simulink model "panelMotor_data_control_2018"  (R2018a)
settings: Solver=VariableStepAuto  StartTime=0.0  StopTime=15*3600  RelTol=1e-3
values from neighbouring files (symbols this model uses):
  J = m/12*(l^2*cos(beta)^2+d^2*sin(beta)^2+w^2)    [panelMotorParams.m]
  Jp = m/12*(w^2*cos(beta)^2+d^2*sin(beta)^2+l^2)    [panelMotorParams.m]
  Kd = 5    [panelMotorParams.m]
  Kf = 0.07    [panelMotorParams.m]
  Kg = 2000    [panelMotorParams.m]
  Kt = 0.07    [panelMotorParams.m]
  L = 1e-5    (= 1e-05)    [panelMotorParams.m]
  R = 10    [panelMotorParams.m]
libraries: simulink x3
settings Model: Creator=goku-ubuntu  LastModifiedBy=goku-ubuntu
settings DataIOCC: ExternalInput=[sunTime, sunPosition, sunElevation]  LoadExternalInput=on

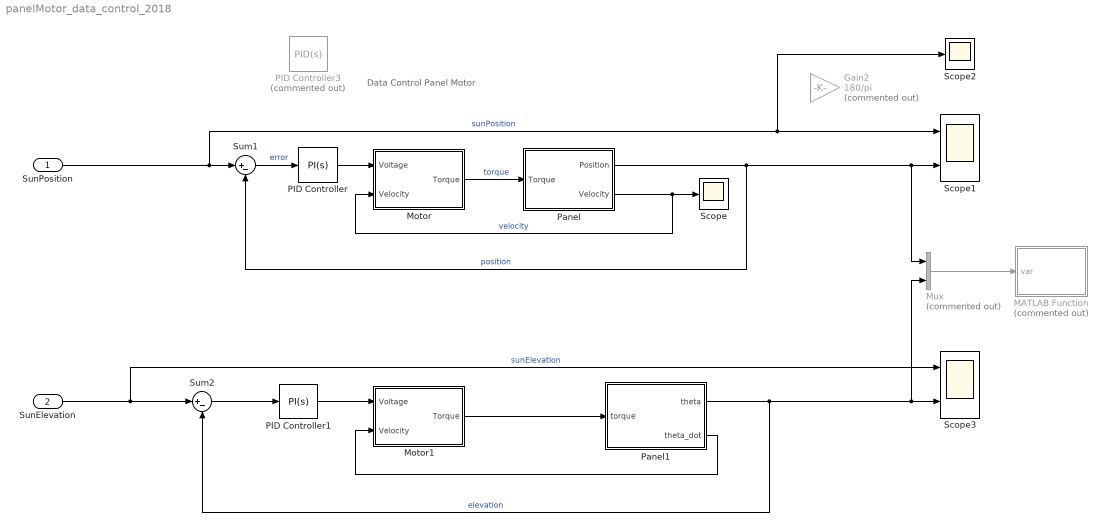
== system panelMotor_data_control_2018 ==
  note: Data Control Panel Motor
  SunPosition : Inport
  SunElevation : Inport  Port=2
  Gain2 : Gain  Commented=on  Gain=180/pi
  MATLAB Function : MATLAB Function  Commented=on  TreatAsAtomicUnit=on
  Motor : Subsystem
  Motor1 : Subsystem
  Mux : Mux  Commented=on  Inputs=2
  PID Controller : simulink/Continuous/PID Controller  Controller=PI  TimeDomain=Continuous-time  SampleTime=-1  IntegratorMethod=Forward Euler  FilterMethod=Forward Euler  Form=Parallel  UseFilter=on  ControllerParametersSource=internal  P=240  I=180  D=0  N=100  InitialConditionSource=internal  InitialConditionForIntegrator=0  InitialConditionForFilter=0  ExternalReset=none  LimitOutput=off  UpperSaturationLimit=inf  LowerSaturationLimit=-inf  LinearizeAsGain=on  AntiWindupMode=none  Kb=1  TrackingMode=off  Kt=1  PParamMin=[]  PParamMax=[]  IParamMin=[]  IParamMax=[]  DParamMin=[]  DParamMax=[]  NParamMin=[]  NParamMax=[]  KbParamMin=[]  KbParamMax=[]  KtParamMin=[]  KtParamMax=[]  POutMin=[]  POutMax=[]  IOutMin=[]  IOutMax=[]  DOutMin=[]  DOutMax=[]  NOutMin=[]  NOutMax=[]  KbOutMin=[]  KbOutMax=[]  KtOutMin=[]  KtOutMax=[]  IntegratorOutMin=[]  IntegratorOutMax=[]  FilterOutMin=[]  FilterOutMax=[]  SumOutMin=[]  SumOutMax=[]  SumI1OutMin=[]  SumI1OutMax=[]  SumI2OutMin=[]  SumI2OutMax=[]  SumI3OutMin=[]  SumI3OutMax=[]  SumDOutMin=[]  SumDOutMax=[]  SaturationOutMin=[]  SaturationOutMax=[]  IntegratorContinuousStateAttributes=''  IntegratorStateMustResolveToSignalObject=off  IntegratorRTWStateStorageClass=Auto  FilterContinuousStateAttributes=''  FilterStateMustResolveToSignalObject=off  FilterRTWStateStorageClass=Auto  DifferentiatorICPrevScaledInput=0  DifferentiatorOutMin=[]  DifferentiatorOutMax=[]  FilterDiffOutCoefMin=[]  FilterDiffOutCoefMax=[]  SumDenOutMin=[]  SumDenOutMax=[]  SumNumOutMin=[]  SumNumOutMax=[]  ReciprocalOutMin=[]  ReciprocalOutMax=[]  DivideOutMin=[]  DivideOutMax=[]  TunerSelectOption=Transfer Function Based (PID Tuner App)
  PID Controller1 : simulink/Continuous/PID Controller  Controller=PI  TimeDomain=Continuous-time  SampleTime=-1  IntegratorMethod=Forward Euler  FilterMethod=Forward Euler  Form=Parallel  UseFilter=on  ControllerParametersSource=internal  P=8839.69591986541  I=114833.219838399  D=0  N=100  InitialConditionSource=internal  InitialConditionForIntegrator=0  InitialConditionForFilter=0  ExternalReset=none  LimitOutput=off  UpperSaturationLimit=inf  LowerSaturationLimit=-inf  LinearizeAsGain=on  AntiWindupMode=none  Kb=1  TrackingMode=off  Kt=1  PParamMin=[]  PParamMax=[]  IParamMin=[]  IParamMax=[]  DParamMin=[]  DParamMax=[]  NParamMin=[]  NParamMax=[]  KbParamMin=[]  KbParamMax=[]  KtParamMin=[]  KtParamMax=[]  POutMin=[]  POutMax=[]  IOutMin=[]  IOutMax=[]  DOutMin=[]  DOutMax=[]  NOutMin=[]  NOutMax=[]  KbOutMin=[]  KbOutMax=[]  KtOutMin=[]  KtOutMax=[]  IntegratorOutMin=[]  IntegratorOutMax=[]  FilterOutMin=[]  FilterOutMax=[]  SumOutMin=[]  SumOutMax=[]  SumI1OutMin=[]  SumI1OutMax=[]  SumI2OutMin=[]  SumI2OutMax=[]  SumI3OutMin=[]  SumI3OutMax=[]  SumDOutMin=[]  SumDOutMax=[]  SaturationOutMin=[]  SaturationOutMax=[]  IntegratorContinuousStateAttributes=''  IntegratorStateMustResolveToSignalObject=off  IntegratorRTWStateStorageClass=Auto  FilterContinuousStateAttributes=''  FilterStateMustResolveToSignalObject=off  FilterRTWStateStorageClass=Auto  DifferentiatorICPrevScaledInput=0  DifferentiatorOutMin=[]  DifferentiatorOutMax=[]  FilterDiffOutCoefMin=[]  FilterDiffOutCoefMax=[]  SumDenOutMin=[]  SumDenOutMax=[]  SumNumOutMin=[]  SumNumOutMax=[]  ReciprocalOutMin=[]  ReciprocalOutMax=[]  DivideOutMin=[]  DivideOutMax=[]  TunerSelectOption=Transfer Function Based (PID Tuner App)
  PID Controller3 : simulink/Continuous/PID Controller  Commented=on  Controller=PID  TimeDomain=Continuous-time  SampleTime=-1  IntegratorMethod=Forward Euler  FilterMethod=Forward Euler  Form=Parallel  UseFilter=on  ControllerParametersSource=internal  P=65852.2280611086  I=3527604.18786694  D=217.337883352011  N=1464.14190878137  InitialConditionSource=internal  InitialConditionForIntegrator=0  InitialConditionForFilter=0  ExternalReset=none  LimitOutput=off  UpperSaturationLimit=inf  LowerSaturationLimit=-inf  LinearizeAsGain=on  AntiWindupMode=none  Kb=1  TrackingMode=off  Kt=1  PParamMin=[]  PParamMax=[]  IParamMin=[]  IParamMax=[]  DParamMin=[]  DParamMax=[]  NParamMin=[]  NParamMax=[]  KbParamMin=[]  KbParamMax=[]  KtParamMin=[]  KtParamMax=[]  POutMin=[]  POutMax=[]  IOutMin=[]  IOutMax=[]  DOutMin=[]  DOutMax=[]  NOutMin=[]  NOutMax=[]  KbOutMin=[]  KbOutMax=[]  KtOutMin=[]  KtOutMax=[]  IntegratorOutMin=[]  IntegratorOutMax=[]  FilterOutMin=[]  FilterOutMax=[]  SumOutMin=[]  SumOutMax=[]  SumI1OutMin=[]  SumI1OutMax=[]  SumI2OutMin=[]  SumI2OutMax=[]  SumI3OutMin=[]  SumI3OutMax=[]  SumDOutMin=[]  SumDOutMax=[]  SaturationOutMin=[]  SaturationOutMax=[]  IntegratorContinuousStateAttributes=''  IntegratorStateMustResolveToSignalObject=off  IntegratorRTWStateStorageClass=Auto  FilterContinuousStateAttributes=''  FilterStateMustResolveToSignalObject=off  FilterRTWStateStorageClass=Auto  DifferentiatorICPrevScaledInput=0  DifferentiatorOutMin=[]  DifferentiatorOutMax=[]  FilterDiffOutCoefMin=[]  FilterDiffOutCoefMax=[]  SumDenOutMin=[]  SumDenOutMax=[]  SumNumOutMin=[]  SumNumOutMax=[]  ReciprocalOutMin=[]  ReciprocalOutMax=[]  DivideOutMin=[]  DivideOutMax=[]  TunerSelectOption=Transfer Function Based (PID Tuner App)
  Panel : Subsystem
  Panel1 : Subsystem
  Scope : Scope
  Scope1 : Scope  NumInputPorts=2
  Scope2 : Scope
  Scope3 : Scope  NumInputPorts=2
  Sum1 : Sum  Inputs=|+-
  Sum2 : Sum  Inputs=|+-
  wires:
  Panel/2(Velocity) -> Motor/2(Velocity), Scope/1  "velocity"
  Panel/1(Position) -> Sum1/2, Mux/1, Scope1/2  "position"
  Motor/1(Torque) -> Panel/1(Torque)  "torque"
  Sum1/1 -> PID Controller/1  "error"
  PID Controller/1 -> Motor/1(Voltage)
  SunPosition/1 -> Sum1/1, Scope1/1, Scope2/1  "sunPosition"
  Motor1/1(Torque) -> Panel1/1(torque)
  Panel1/2(theta_dot) -> Motor1/2(Velocity)
  Panel1/1(theta) -> Sum2/2, Mux/2, Scope3/2  "elevation"
  PID Controller1/1 -> Motor1/1(Voltage)
  Sum2/1 -> PID Controller1/1
  SunElevation/1 -> Sum2/1, Scope3/1  "sunElevation"
  Mux/1 -> MATLAB Function/1(var)

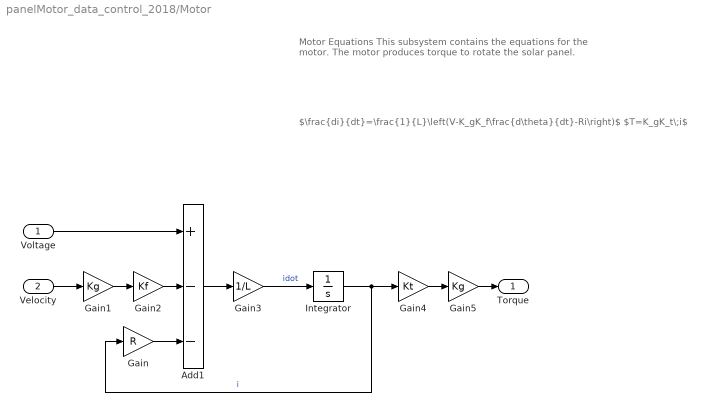
== system panelMotor_data_control_2018/Motor ==
  note: $\frac{di}{dt}=\frac{1}{L}\left(V-K_gK_f\frac{d\theta}{dt}-Ri\right)$
      | $T=K_gK_t\;i$
  note: Motor Equations
      |
      | This subsystem contains the equations for the motor. The motor produces torque to rotate the solar panel.
  Voltage : Inport
  Velocity : Inport  Port=2
  Add1 : Sum  Inputs=+--
  Gain : Gain  Gain=R
  Gain1 : Gain  Gain=Kg
  Gain2 : Gain  Gain=Kf
  Gain3 : Gain  Gain=1/L
  Gain4 : Gain  Gain=Kt
  Gain5 : Gain  Gain=Kg
  Integrator : Integrator
  Torque : Outport  VectorParamsAs1DForOutWhenUnconnected=on
  wires:
  Voltage/1 -> Add1/1
  Gain2/1 -> Add1/2
  Gain3/1 -> Integrator/1  "idot"
  Gain/1 -> Add1/3
  Integrator/1 -> Gain4/1, Gain/1  "i"
  Add1/1 -> Gain3/1
  Velocity/1 -> Gain1/1
  Gain4/1 -> Gain5/1
  Gain1/1 -> Gain2/1
  Gain5/1 -> Torque/1

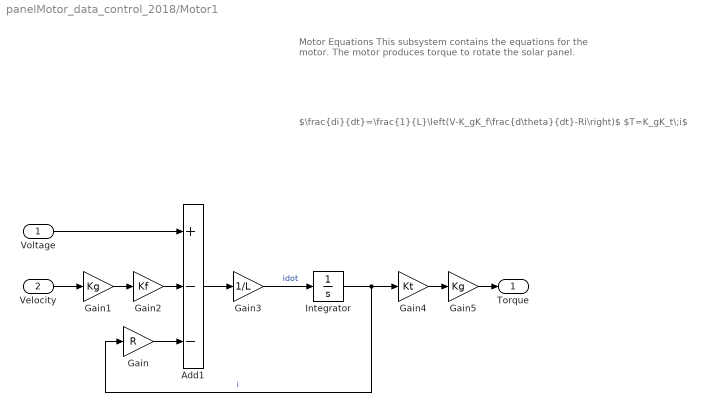
== system panelMotor_data_control_2018/Motor1 ==
  note: Motor Equations
      |
      | This subsystem contains the equations for the motor. The motor produces torque to rotate the solar panel.
  note: $\frac{di}{dt}=\frac{1}{L}\left(V-K_gK_f\frac{d\theta}{dt}-Ri\right)$
      | $T=K_gK_t\;i$
  Voltage : Inport
  Velocity : Inport  Port=2
  Add1 : Sum  Inputs=+--
  Gain : Gain  Gain=R
  Gain1 : Gain  Gain=Kg
  Gain2 : Gain  Gain=Kf
  Gain3 : Gain  Gain=1/L
  Gain4 : Gain  Gain=Kt
  Gain5 : Gain  Gain=Kg
  Integrator : Integrator
  Torque : Outport  VectorParamsAs1DForOutWhenUnconnected=on
  wires:
  Gain5/1 -> Torque/1
  Gain1/1 -> Gain2/1
  Gain4/1 -> Gain5/1
  Velocity/1 -> Gain1/1
  Add1/1 -> Gain3/1
  Integrator/1 -> Gain/1, Gain4/1  "i"
  Gain/1 -> Add1/3
  Gain3/1 -> Integrator/1  "idot"
  Gain2/1 -> Add1/2
  Voltage/1 -> Add1/1

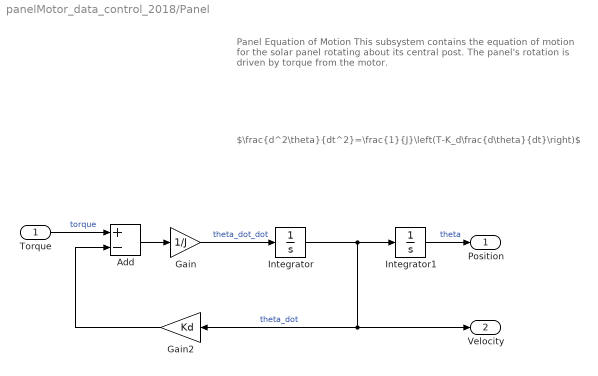
== system panelMotor_data_control_2018/Panel ==
  note: $\frac{d^2\theta}{dt^2}=\frac{1}{J}\left(T-K_d\frac{d\theta}{dt}\right)$
  note: Panel Equation of Motion
      |
      | This subsystem contains the equation of motion for the solar panel rotating about its central post. The panel's rotation is driven by torque from the motor.
  Torque : Inport
  Add : Sum  Inputs=+-
  Gain : Gain  Gain=1/J
  Gain2 : Gain  Gain=Kd
  Integrator : Integrator
  Integrator1 : Integrator
  Position : Outport  VectorParamsAs1DForOutWhenUnconnected=on
  Velocity : Outport  Port=2  VectorParamsAs1DForOutWhenUnconnected=on
  wires:
  Torque/1 -> Add/1  "torque"
  Add/1 -> Gain/1
  Integrator/1 -> Integrator1/1, Velocity/1, Gain2/1  "theta_dot"
  Gain2/1 -> Add/2
  Gain/1 -> Integrator/1  "theta_dot_dot"
  Integrator1/1 -> Position/1  "theta"

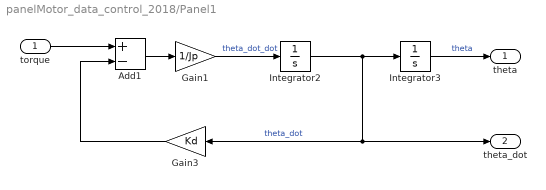
== system panelMotor_data_control_2018/Panel1 ==
  torque : Inport
  Add1 : Sum  Inputs=+-
  Gain1 : Gain  Gain=1/Jp
  Gain3 : Gain  Gain=Kd
  Integrator2 : Integrator
  Integrator3 : Integrator
  theta : Outport
  theta_dot : Outport  Port=2
  wires:
  Gain1/1 -> Integrator2/1  "theta_dot_dot"
  Gain3/1 -> Add1/2
  Add1/1 -> Gain1/1
  Integrator3/1 -> theta/1  "theta"
  Integrator2/1 -> Integrator3/1, theta_dot/1, Gain3/1  "theta_dot"
  torque/1 -> Add1/1

== matlab function panelMotor_data_control_2018/MATLAB Function ==
  data: var input
function fcn(var)

position = var(0);
elevation = var(1);

plot3(sunTime, rad2deg(position), rad2deg(elevation))
